simulink subsystem "Nitrous_Tank_Custom"  (R2020b)
settings: Solver=VariableStepAuto  StartTime=0.0  StopTime=10.0  RelTol=1e-3
model mask{nitrousLiqConCrossSection=3.8485e-05, nitrousVapConCrossSection=2e-5, nitrousTankVol=0.0141, initialTankPressure=60e5, initialLiqMassFraction=0.7, totalHeatTransferSurfaceArea=6, heatTranferWallToLiq=0, heatTranferWallToVap=0}
  mask prompts: nitrousLiqConCrossSection "Liquid port cross section in m^2"; nitrousVapConCrossSection "Vapour port cross section in m^2"; nitrousTankVol "Tank Volume in m^3"; initialTankPressure "Tank start pressure in Pa"; initialLiqMassFraction "Fraction of the nitrous in the tank which starts out liquid (By mass)"; totalHeatTransferSurfaceArea "Total heat transfer surface area (inner wall) m^2"; heatTranferWallToLiq "Heat transfer coefficient wall to liquid"; heatTranferWallToVap "Heat transfer coefficient wall to vapour"
libraries: nesl_utility x5, fl_lib x2, SimscapeCustomBlocks_lib x2
(part 2 of 2)

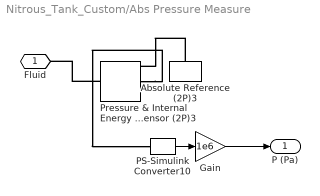
== system Nitrous_Tank_Custom/Abs Pressure Measure ==
  Absolute Reference (2P)3 : fl_lib/Two-Phase Fluid/Elements/Absolute Reference (2P)
      settings: SourceProductBaseCode=SS
  Gain : Gain  Gain=1e6
  PS-Simulink Converter10 : nesl_utility/PS-Simulink Converter  PhysicalDomain=network_engine_domain  SubClassName=ps_output  LeftPortType=input  RightPortType=output  PseudoPeriodic=off  Frequencies=[]  Unit=inherit  AffineConversion=off
  Pressure & Internal Energy Sensor (2P)3 : fl_lib/Two-Phase Fluid/Sensors/Pressure & Internal Energy Sensor (2P)
      settings: SourceProductBaseCode=SS  InternalSimscapePortConfiguration="{\"Bottom\":[],\"Left\":[{\"id\":\"A\",\"label\":\"A\",\"type\":\"foundation.two_phase_fluid.two_phase_fluid\"}],\"Right\":[{\"id\":\"B\",\"label\":\"B\",\"type\":\"foundation.two_phase_fluid.two_phase_fluid\"},{\"id\":\"P\",\"label\":\"P\",\"type\":\"output\"},{\"id\":\"U\",\"label\":\"U\",\"type\":\"output\"}],\"Top\":[]}"
  Fluid : PMIOPort  Side=Left
  P (Pa) : Outport
  wires:
  Gain/1 -> P (Pa)/1
  PS-Simulink Converter10/1 -> Gain/1
  connections:
  Pressure & Internal Energy Sensor (2P)3/LConn1 -- Fluid/RConn1
  Pressure & Internal Energy Sensor (2P)3/RConn2 -- PS-Simulink Converter10/LConn1
  Absolute Reference (2P)3/LConn1 -- Pressure & Internal Energy Sensor (2P)3/RConn1
